simulink library "relay_ANSI_functions_lib"  (Simulink 8.1)
settings: Solver=ode45  StartTime=0.0  StopTime=10.0  RelTol=1e-3
undefined symbols (not defined in the file or in its folder): DiscIntNeverNeededParam, IOC, TOC, Ts, VRMSLL
libraries: simulink x8
settings Model: Creator=RE25624  LastModifiedBy=hptb1

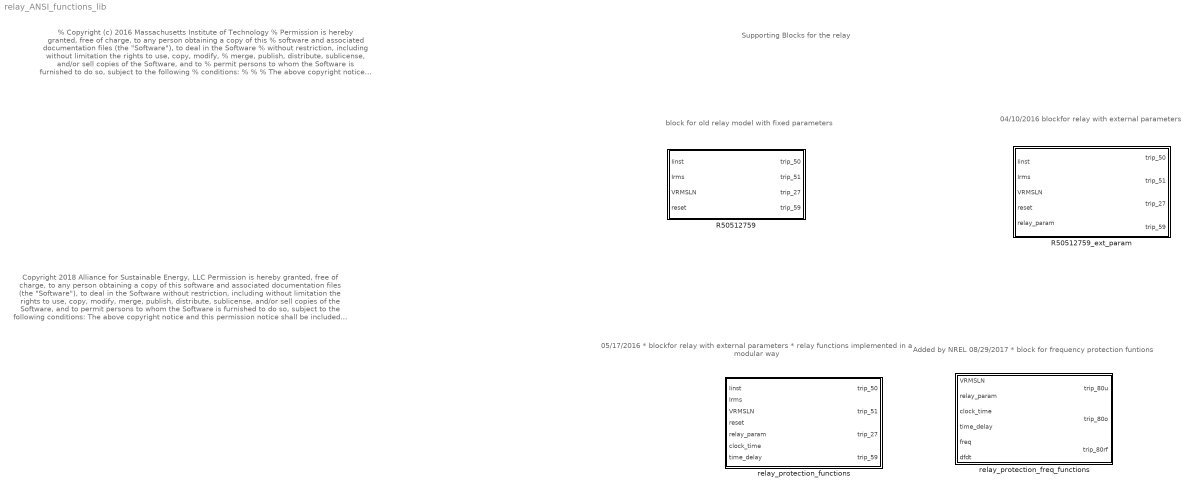
== system relay_ANSI_functions_lib ==
  note: 04/10/2016
      | blockfor relay with external parameters
  note: Supporting Blocks for the relay
  note: block for old relay model with fixed parameters
  note: 05/17/2016
      | * blockfor relay with external parameters
      | * relay functions implemented in a modular way
  note: % Copyright (c) 2016 Massachusetts Institute of Technology
      | % Permission is hereby granted, free of charge, to any person obtaining a copy of this
      | % software and associated documentation files (the "Software"), to deal in the Software
      | % without restriction, including without limitation the rights to use, copy, modify,
      | % merge, publish, distribute, sublicense, and/or sell copies of the Software, and to
      | % permit persons to whom the Software is furnished to do so, subject to the following
      | % conditions:
      | %
      | %
      | % The above copyright notice and this permission notice shall be included in
      | % all copies or substantial portions of the Software.
      | %
      | % THE SOFTWARE IS PROVIDED "AS IS", WITHOUT WARRANTY OF ANY KIND, EXPRESS OR IMPLIED,
      | % INCLUDING BUT NOT LIMITED TO THE WARRANTIES OF MERCHANTABILITY, FITNESS FOR A
      | % PARTICULAR PURPOSE AND NONINFRINGEMENT. IN NO EVENT SHALL THE AUTHORS OR COPYRIGHT
      | % HOLDERS BE LIABLE FOR ANY CLAIM, DAMAGES OR OTHER LIABILITY, WHETHER IN AN ACTION
      | % OF CONTRACT, TORT OR OTHERWISE, ARISING FROM, OUT OF OR IN CONNECTION WITH THE
      | % SOFTWARE OR THE USE OR OTHER DEALINGS IN THE SOFTWARE.
      | %
      | %
      | %%
  note: Added by NREL 08/29/2017
      | * block for frequency protection funtions
  note: Copyright 2018 Alliance for Sustainable Energy, LLC
      |
      | Permission is hereby granted, free of charge, to any person obtaining a copy of this software
      | and associated documentation files (the "Software"), to deal in the Software without restriction,
      | including without limitation the rights to use, copy, modify, merge, publish, distribute, sublicense,
      | and/or sell copies of the Software, and to permit persons to whom the Software is furnished to do so,
      | subject to the following conditions:
      |
      | The above copyright notice and this permission notice shall be included in all copies or substantial portions of the Software.
      |
      | THE SOFTWARE IS PROVIDED "AS IS", WITHOUT WARRANTY OF ANY KIND, EXPRESS OR IMPLIED, INCLUDING
      | BUT NOT LIMITED TO THE WARRANTIES OF MERCHANTABILITY, FITNESS FOR A PARTICULAR PURPOSE AND
      | NONINFRINGEMENT. IN NO EVENT SHALL THE AUTHORS, THE COPYRIGHT HOLDERS, THE UNITED STATES,
      | THE UNITED STATES DEPARTMENT OF ENERGY, OR ANY OF THEIR EMPLOYEES BE LIABLE FOR ANY CLAIM,
      | DAMAGES OR OTHER LIABILITY, WHETHER IN AN ACTION OF CONTRACT, TORT OR OTHERWISE, ARISING FROM,
      | OUT OF OR IN CONNECTION WITH THE SOFTWARE OR THE USE OR OTHER DEALINGS IN THE SOFTWARE.
  R50512759 : Subsystem  mask(Relays 50-51-27-59){VRMSLL=VRMSLL, IOC=IOC, TOC=TOC, Ts=Ts}
      mask prompts: VRMSLL "Nominal Voltage [VRMSLL]"; IOC "IOC Setting [A]"; TOC "TOC Setting [A]"; Ts "Sampling Time [Sec]"
      mask help:
      | This block simulates the behavior of the following relay functions:
      | 1) Instantaneous overcurrent (50)
      | 2) AC inverse time overcurrent (51)
      | 3) Undervoltage (27)
      | 4) Overvoltage (59)
      | It is not suitable for instantaneous earth current relaying.
      | The model neglects the influence CTs since only the logics of the relay are required or the current effort.
  R50512759_ext_param : Subsystem  mask(Relays 50-51-27-59){Ts=Ts}
      mask prompts: Ts "Sampling Time [Sec]"
      mask help:
      | This block simulates the behavior of the following relay functions:
      | 1) Instantaneous overcurrent (50)
      | 2) AC inverse time overcurrent (51)
      | 3) Undervoltage (27)
      | 4) Overvoltage (59)
      | It is not suitable for instantaneous earth current relaying.
      | The model neglects the influence CTs since only the logics of the relay are required or the current effort.
      |
      | The input bus with the relay parameters should be ordered as follows:
      | 1) VRMSLL
      | 2) IOC
      | 3) TOC
      | 4) dV_threshold
      | 5) angle_threshold
      | 6) dF_threshold
  relay_protection_freq_functions : Subsystem  mask(Relays 50-51-27-59){Ts=Ts}
      mask prompts: Ts "Sampling Time [Sec]"
      mask help:
      | This block simulates the behavior of the following relay functions:
      | 1)	Overfrequency (ANSI 81O)
      | 2)	Underfrequency (ANSI 81U)
      | 3)	Fast rate of change of frequency (ANSI 81R)
  relay_protection_functions : Subsystem  mask(Relays 50-51-27-59){Ts=Ts}
      mask prompts: Ts "Sampling Time [Sec]"
      mask help:
      | This block simulates the behavior of the following relay functions:
      | 1) Instantaneous overcurrent (50)
      | 2) AC inverse time overcurrent (51)
      | 3) Undervoltage (27)
      | 4) Overvoltage (59)
      | It is not suitable for instantaneous earth current relaying.
      | The model neglects the influence CTs since only the logics of the relay are required or the current effort.
      |
      | The input bus with the relay parameters should be ordered as follows:
      | 1) VRMSLL
      | 2) IOC
      | 3) TOC
      | 4) dV_threshold
      | 5) angle_threshold
      | 6) dF_threshold

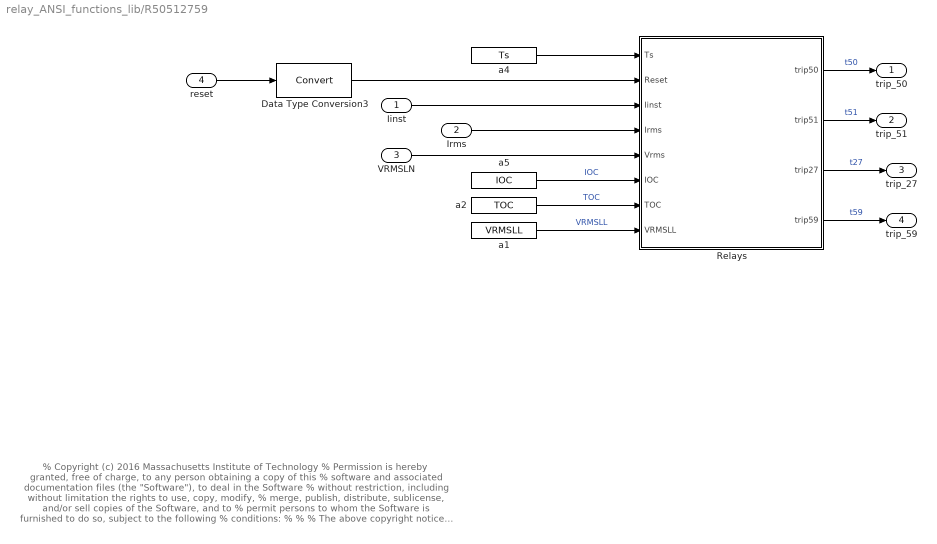
== system relay_ANSI_functions_lib/R50512759 ==
  note: % Copyright (c) 2016 Massachusetts Institute of Technology
      | % Permission is hereby granted, free of charge, to any person obtaining a copy of this
      | % software and associated documentation files (the "Software"), to deal in the Software
      | % without restriction, including without limitation the rights to use, copy, modify,
      | % merge, publish, distribute, sublicense, and/or sell copies of the Software, and to
      | % permit persons to whom the Software is furnished to do so, subject to the following
      | % conditions:
      | %
      | %
      | % The above copyright notice and this permission notice shall be included in
      | % all copies or substantial portions of the Software.
      | %
      | % THE SOFTWARE IS PROVIDED "AS IS", WITHOUT WARRANTY OF ANY KIND, EXPRESS OR IMPLIED,
      | % INCLUDING BUT NOT LIMITED TO THE WARRANTIES OF MERCHANTABILITY, FITNESS FOR A
      | % PARTICULAR PURPOSE AND NONINFRINGEMENT. IN NO EVENT SHALL THE AUTHORS OR COPYRIGHT
      | % HOLDERS BE LIABLE FOR ANY CLAIM, DAMAGES OR OTHER LIABILITY, WHETHER IN AN ACTION
      | % OF CONTRACT, TORT OR OTHERWISE, ARISING FROM, OUT OF OR IN CONNECTION WITH THE
      | % SOFTWARE OR THE USE OR OTHER DEALINGS IN THE SOFTWARE.
      | %
      | %
      | %%
  Iinst : Inport
  Irms : Inport  Port=2
  VRMSLN : Inport  Port=3
  reset : Inport  Port=4
  Data Type Conversion3 : DataTypeConversion
  Relays : MATLAB Function  TreatAsAtomicUnit=on
  a1 : Constant  Value=VRMSLL
  a2 : Constant  Value=TOC
  a4 : Constant  Value=Ts
  a5 : Constant  Value=IOC
  trip_50 : Outport
  trip_51 : Outport  Port=2
  trip_27 : Outport  Port=3
  trip_59 : Outport  Port=4
  wires:
  Data Type Conversion3/1 -> Relays/2(Reset)
  Relays/2(trip51) -> trip_51/1  "t51"
  Relays/1(trip50) -> trip_50/1  "t50"
  Relays/4(trip59) -> trip_59/1  "t59"
  Relays/3(trip27) -> trip_27/1  "t27"
  a4/1 -> Relays/1(Ts)
  a1/1 -> Relays/8(VRMSLL)  "VRMSLL"
  VRMSLN/1 -> Relays/5(Vrms)
  Irms/1 -> Relays/4(Irms)
  a2/1 -> Relays/7(TOC)  "TOC"
  Iinst/1 -> Relays/3(Iinst)
  a5/1 -> Relays/6(IOC)  "IOC"
  reset/1 -> Data Type Conversion3/1

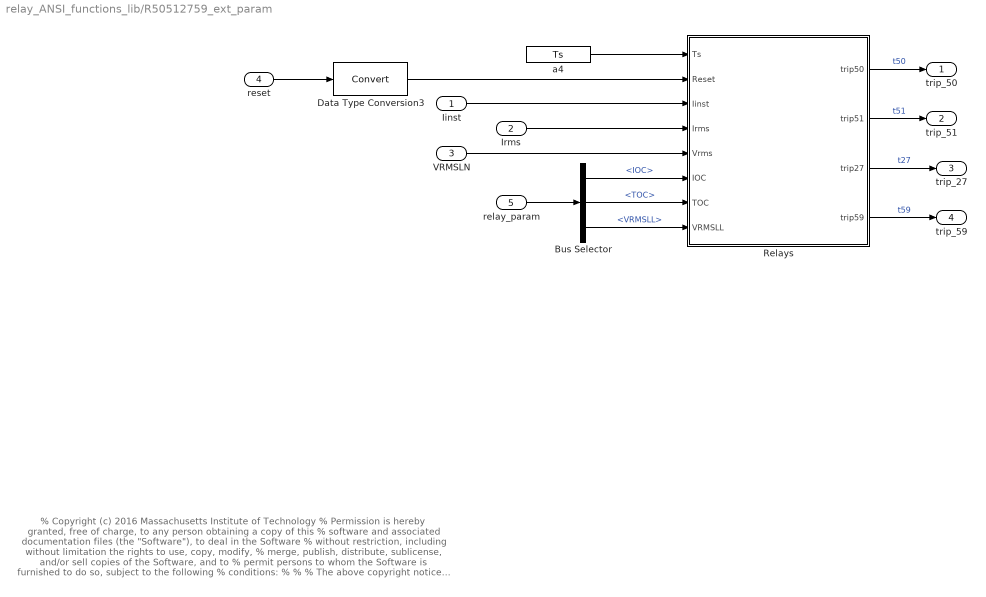
== system relay_ANSI_functions_lib/R50512759_ext_param ==
  note: % Copyright (c) 2016 Massachusetts Institute of Technology
      | % Permission is hereby granted, free of charge, to any person obtaining a copy of this
      | % software and associated documentation files (the "Software"), to deal in the Software
      | % without restriction, including without limitation the rights to use, copy, modify,
      | % merge, publish, distribute, sublicense, and/or sell copies of the Software, and to
      | % permit persons to whom the Software is furnished to do so, subject to the following
      | % conditions:
      | %
      | %
      | % The above copyright notice and this permission notice shall be included in
      | % all copies or substantial portions of the Software.
      | %
      | % THE SOFTWARE IS PROVIDED "AS IS", WITHOUT WARRANTY OF ANY KIND, EXPRESS OR IMPLIED,
      | % INCLUDING BUT NOT LIMITED TO THE WARRANTIES OF MERCHANTABILITY, FITNESS FOR A
      | % PARTICULAR PURPOSE AND NONINFRINGEMENT. IN NO EVENT SHALL THE AUTHORS OR COPYRIGHT
      | % HOLDERS BE LIABLE FOR ANY CLAIM, DAMAGES OR OTHER LIABILITY, WHETHER IN AN ACTION
      | % OF CONTRACT, TORT OR OTHERWISE, ARISING FROM, OUT OF OR IN CONNECTION WITH THE
      | % SOFTWARE OR THE USE OR OTHER DEALINGS IN THE SOFTWARE.
      | %
      | %
      | %%
  Iinst : Inport
  Irms : Inport  Port=2
  VRMSLN : Inport  Port=3
  reset : Inport  Port=4
  relay_param : Inport  Port=5
  Bus Selector : BusSelector  OutputSignals=IOC,TOC,VRMSLL
  Data Type Conversion3 : DataTypeConversion
  Relays : MATLAB Function  TreatAsAtomicUnit=on
  a4 : Constant  Value=Ts
  trip_50 : Outport
  trip_51 : Outport  Port=2
  trip_27 : Outport  Port=3
  trip_59 : Outport  Port=4
  wires:
  relay_param/1 -> Bus Selector/1
  Data Type Conversion3/1 -> Relays/2(Reset)
  Relays/2(trip51) -> trip_51/1  "t51"
  Relays/1(trip50) -> trip_50/1  "t50"
  Relays/4(trip59) -> trip_59/1  "t59"
  Relays/3(trip27) -> trip_27/1  "t27"
  a4/1 -> Relays/1(Ts)
  Bus Selector/3 -> Relays/8(VRMSLL)  "<VRMSLL>"
  VRMSLN/1 -> Relays/5(Vrms)
  Irms/1 -> Relays/4(Irms)
  Bus Selector/2 -> Relays/7(TOC)  "<TOC>"
  Iinst/1 -> Relays/3(Iinst)
  Bus Selector/1 -> Relays/6(IOC)  "<IOC>"
  reset/1 -> Data Type Conversion3/1

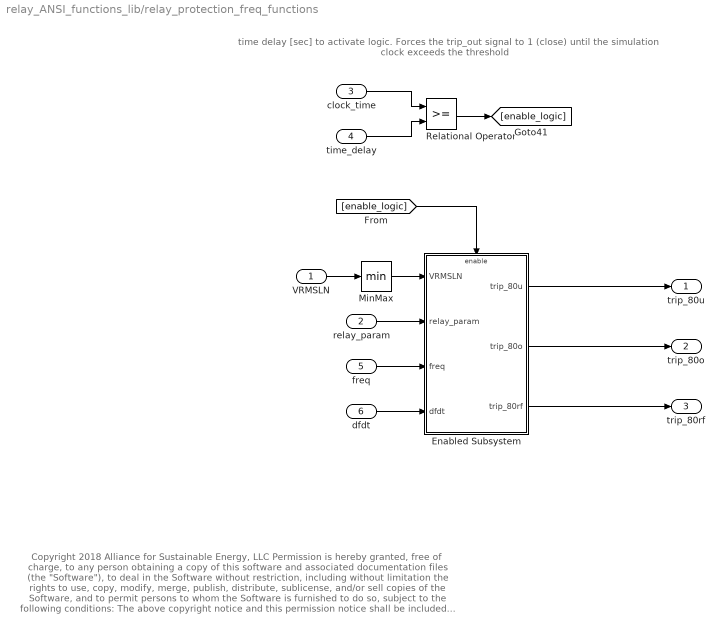
== system relay_ANSI_functions_lib/relay_protection_freq_functions ==
  note: Copyright 2018 Alliance for Sustainable Energy, LLC
      |
      | Permission is hereby granted, free of charge, to any person obtaining a copy of this software
      | and associated documentation files (the "Software"), to deal in the Software without restriction,
      | including without limitation the rights to use, copy, modify, merge, publish, distribute, sublicense,
      | and/or sell copies of the Software, and to permit persons to whom the Software is furnished to do so,
      | subject to the following conditions:
      |
      | The above copyright notice and this permission notice shall be included in all copies or substantial portions of the Software.
      |
      | THE SOFTWARE IS PROVIDED "AS IS", WITHOUT WARRANTY OF ANY KIND, EXPRESS OR IMPLIED, INCLUDING
      | BUT NOT LIMITED TO THE WARRANTIES OF MERCHANTABILITY, FITNESS FOR A PARTICULAR PURPOSE AND
      | NONINFRINGEMENT. IN NO EVENT SHALL THE AUTHORS, THE COPYRIGHT HOLDERS, THE UNITED STATES,
      | THE UNITED STATES DEPARTMENT OF ENERGY, OR ANY OF THEIR EMPLOYEES BE LIABLE FOR ANY CLAIM,
      | DAMAGES OR OTHER LIABILITY, WHETHER IN AN ACTION OF CONTRACT, TORT OR OTHERWISE, ARISING FROM,
      | OUT OF OR IN CONNECTION WITH THE SOFTWARE OR THE USE OR OTHER DEALINGS IN THE SOFTWARE.
  note: time delay [sec] to activate logic. Forces the trip_out signal
      | to 1 (close) until the simulation clock exceeds the threshold
  VRMSLN : Inport
  relay_param : Inport  Port=2
  clock_time : Inport  Port=3
  time_delay : Inport  Port=4
  freq : Inport  Port=5
  dfdt : Inport  Port=6
  Enabled Subsystem : Subsystem  TreatAsAtomicUnit=on
  MinMax : MinMax
  Relational Operator : RelationalOperator  OutDataTypeStr=boolean
  trip_80u : Outport
  trip_80o : Outport  Port=2
  trip_80rf : Outport  Port=3
  wires:
  [enable_logic] -> Enabled Subsystem/Enable
  Relational Operator/1 -> [enable_logic]
  time_delay/1 -> Relational Operator/2
  clock_time/1 -> Relational Operator/1
  VRMSLN/1 -> MinMax/1
  Enabled Subsystem/1(trip_80u) -> trip_80u/1
  Enabled Subsystem/2(trip_80o) -> trip_80o/1
  Enabled Subsystem/3(trip_80rf) -> trip_80rf/1
  relay_param/1 -> Enabled Subsystem/2(relay_param)
  freq/1 -> Enabled Subsystem/3(freq)
  dfdt/1 -> Enabled Subsystem/4(dfdt)
  MinMax/1 -> Enabled Subsystem/1(VRMSLN)

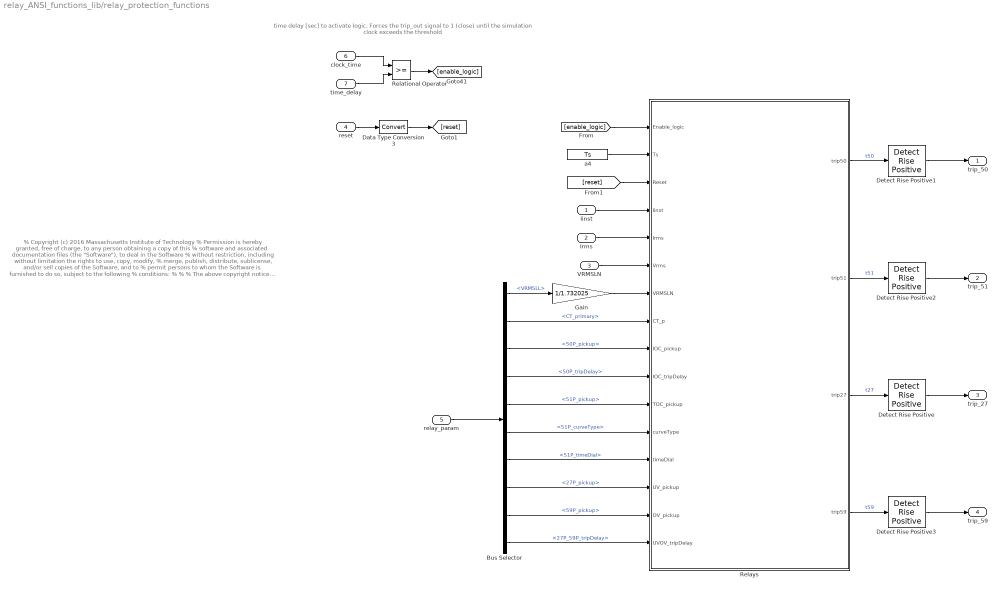
== system relay_ANSI_functions_lib/relay_protection_functions ==
  note: % Copyright (c) 2016 Massachusetts Institute of Technology
      | % Permission is hereby granted, free of charge, to any person obtaining a copy of this
      | % software and associated documentation files (the "Software"), to deal in the Software
      | % without restriction, including without limitation the rights to use, copy, modify,
      | % merge, publish, distribute, sublicense, and/or sell copies of the Software, and to
      | % permit persons to whom the Software is furnished to do so, subject to the following
      | % conditions:
      | %
      | %
      | % The above copyright notice and this permission notice shall be included in
      | % all copies or substantial portions of the Software.
      | %
      | % THE SOFTWARE IS PROVIDED "AS IS", WITHOUT WARRANTY OF ANY KIND, EXPRESS OR IMPLIED,
      | % INCLUDING BUT NOT LIMITED TO THE WARRANTIES OF MERCHANTABILITY, FITNESS FOR A
      | % PARTICULAR PURPOSE AND NONINFRINGEMENT. IN NO EVENT SHALL THE AUTHORS OR COPYRIGHT
      | % HOLDERS BE LIABLE FOR ANY CLAIM, DAMAGES OR OTHER LIABILITY, WHETHER IN AN ACTION
      | % OF CONTRACT, TORT OR OTHERWISE, ARISING FROM, OUT OF OR IN CONNECTION WITH THE
      | % SOFTWARE OR THE USE OR OTHER DEALINGS IN THE SOFTWARE.
      | %
      | %
      | %%
  note: time delay [sec] to activate logic. Forces the trip_out signal
      | to 1 (close) until the simulation clock exceeds the threshold
  Iinst : Inport
  Irms : Inport  Port=2
  VRMSLN : Inport  Port=3
  reset : Inport  Port=4
  relay_param : Inport  Port=5
  clock_time : Inport  Port=6
  time_delay : Inport  Port=7
  Bus Selector : BusSelector  OutputSignals=VRMSLL,CT_primary,50P_pickup,50P_tripDelay,51P_pickup,51P_curveType,51P_timeDial,27P_pickup,59P_pickup,27P_59P_tripDelay
  Data Type Conversion3 : DataTypeConversion
  Detect Rise Positive{,1..3} (4 alike) : simulink/Logic and Bit Operations/Detect Rise Positive  vinit=0  InputProcessing=Inherited  OutDataTypeStr=boolean
  Gain : Gain  Gain=1/1.732025
  Relational Operator : RelationalOperator  OutDataTypeStr=boolean
  Relays : MATLAB Function  TreatAsAtomicUnit=on
  a4 : Constant  Value=Ts
  trip_50 : Outport
  trip_51 : Outport  Port=2
  trip_27 : Outport  Port=3
  trip_59 : Outport  Port=4
  wires:
  [enable_logic] -> Relays/1(Enable_logic)
  Relational Operator/1 -> [enable_logic]
  time_delay/1 -> Relational Operator/2
  clock_time/1 -> Relational Operator/1
  relay_param/1 -> Bus Selector/1
  a4/1 -> Relays/2(Ts)
  VRMSLN/1 -> Relays/6(Vrms)
  reset/1 -> Data Type Conversion3/1
  Bus Selector/1 -> Gain/1  "<VRMSLL>"
  Bus Selector/2 -> Relays/8(CT_p)  "<CT_primary>"
  Bus Selector/3 -> Relays/9(IOC_pickup)  "<50P_pickup>"
  Bus Selector/4 -> Relays/10(IOC_tripDelay)  "<50P_tripDelay>"
  Bus Selector/5 -> Relays/11(TOC_pickup)  "<51P_pickup>"
  Bus Selector/6 -> Relays/12(curveType)  "<51P_curveType>"
  Bus Selector/7 -> Relays/13(timeDial)  "<51P_timeDial>"
  Irms/1 -> Relays/5(Irms)
  Iinst/1 -> Relays/4(Iinst)
  Bus Selector/10 -> Relays/16(UVOV_tripDelay)  "<27P_59P_tripDelay>"
  Bus Selector/9 -> Relays/15(OV_pickup)  "<59P_pickup>"
  Bus Selector/8 -> Relays/14(UV_pickup)  "<27P_pickup>"
  Gain/1 -> Relays/7(VRMSLN)
  Data Type Conversion3/1 -> [reset]
  [reset] -> Relays/3(Reset)
  Relays/3(trip27) -> Detect Rise Positive/1  "t27"
  Relays/1(trip50) -> Detect Rise Positive1/1  "t50"
  Relays/2(trip51) -> Detect Rise Positive2/1  "t51"
  Relays/4(trip59) -> Detect Rise Positive3/1  "t59"
  Detect Rise Positive1/1 -> trip_50/1
  Detect Rise Positive2/1 -> trip_51/1
  Detect Rise Positive/1 -> trip_27/1
  Detect Rise Positive3/1 -> trip_59/1

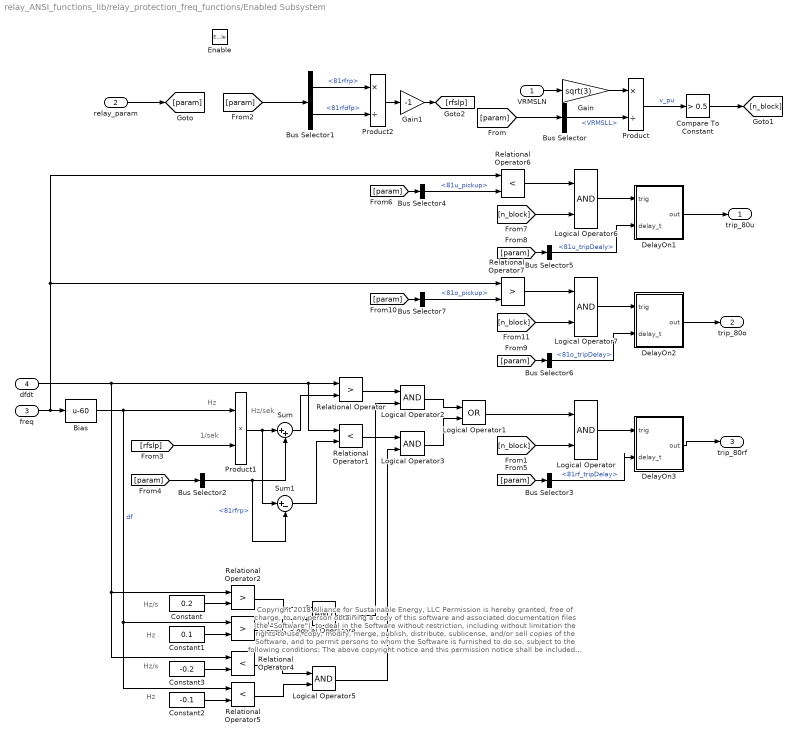
== system relay_ANSI_functions_lib/relay_protection_freq_functions/Enabled Subsystem ==
  note: Copyright 2018 Alliance for Sustainable Energy, LLC
      |
      | Permission is hereby granted, free of charge, to any person obtaining a copy of this software
      | and associated documentation files (the "Software"), to deal in the Software without restriction,
      | including without limitation the rights to use, copy, modify, merge, publish, distribute, sublicense,
      | and/or sell copies of the Software, and to permit persons to whom the Software is furnished to do so,
      | subject to the following conditions:
      |
      | The above copyright notice and this permission notice shall be included in all copies or substantial portions of the Software.
      |
      | THE SOFTWARE IS PROVIDED "AS IS", WITHOUT WARRANTY OF ANY KIND, EXPRESS OR IMPLIED, INCLUDING
      | BUT NOT LIMITED TO THE WARRANTIES OF MERCHANTABILITY, FITNESS FOR A PARTICULAR PURPOSE AND
      | NONINFRINGEMENT. IN NO EVENT SHALL THE AUTHORS, THE COPYRIGHT HOLDERS, THE UNITED STATES,
      | THE UNITED STATES DEPARTMENT OF ENERGY, OR ANY OF THEIR EMPLOYEES BE LIABLE FOR ANY CLAIM,
      | DAMAGES OR OTHER LIABILITY, WHETHER IN AN ACTION OF CONTRACT, TORT OR OTHERWISE, ARISING FROM,
      | OUT OF OR IN CONNECTION WITH THE SOFTWARE OR THE USE OR OTHER DEALINGS IN THE SOFTWARE.
  note: Hz
  note: Hz/sek
  note: 1/sek
  note: Hz
  note: Hz
  note: Hz/s
  note: Hz/s
  VRMSLN : Inport
  relay_param : Inport  Port=2
  freq : Inport  Port=3
  dfdt : Inport  Port=4
  Enable : EnablePort
  Bias : Bias  Bias=-60
  Bus Selector : BusSelector  OutputSignals=VRMSLL
  Bus Selector1 : BusSelector  OutputSignals=81rfrp,81rfdfp
  Bus Selector2 : BusSelector  OutputSignals=81rfrp
  Bus Selector3 : BusSelector  OutputSignals=81rf_tripDelay
  Bus Selector4 : BusSelector  OutputSignals=81u_pickup
  Bus Selector5 : BusSelector  OutputSignals=81u_tripDealy
  Bus Selector6 : BusSelector  OutputSignals=81o_tripDelay
  Bus Selector7 : BusSelector  OutputSignals=81o_pickup
  Compare To Constant : simulink/Logic and Bit Operations/Compare To Constant  relop=>  const=0.5  OutDataTypeStr=boolean
  Constant : Constant  Value=0.2
  Constant1 : Constant  Value=0.1
  Constant2 : Constant  Value=-0.1
  Constant3 : Constant  Value=-0.2
  DelayOn1 : Subsystem
  DelayOn2 : Subsystem
  DelayOn3 : Subsystem
  Gain : Gain  Gain=sqrt(3)
  Gain1 : Gain  Gain=-1
  Logical Operator{,2..7} (7 alike) : Logic  AllPortsSameDT=off  OutDataTypeStr=boolean
  Logical Operator1 : Logic  Operator=OR  AllPortsSameDT=off  OutDataTypeStr=boolean
  Product : Product  Inputs=*/
  Product1 : Product
  Product2 : Product  Inputs=*/
  Relational Operator{,2..3,7} (4 alike) : RelationalOperator  Operator=>  OutDataTypeStr=boolean
  Relational Operator{1,4..6} (4 alike) : RelationalOperator  Operator=<  OutDataTypeStr=boolean
  Sum : Sum  Inputs=|++
  Sum1 : Sum  Inputs=|+-
  trip_80u : Outport
  trip_80o : Outport  Port=2
  trip_80rf : Outport  Port=3
  wires:
  relay_param/1 -> [param]
  [param] -> Bus Selector/1
  VRMSLN/1 -> Gain/1
  Bus Selector/1 -> Product/2  "<VRMSLL>"
  Product/1 -> Compare To Constant/1  "v_pu"
  Gain/1 -> Product/1
  Compare To Constant/1 -> [n_block]
  [n_block] -> Logical Operator/2
  Logical Operator1/1 -> Logical Operator/1
  dfdt/1 -> Relational Operator4/1, Relational Operator2/1, Relational Operator/1, Relational Operator1/1
  [param] -> Bus Selector1/1
  Bus Selector1/1 -> Product2/1  "<81rfrp>"
  freq/1 -> Relational Operator7/1, Relational Operator6/1, Bias/1
  Sum1/1 -> Relational Operator1/2
  Bias/1 -> Relational Operator5/1, Relational Operator3/1, Product1/1  "df"
  [rfslp] -> Product1/2
  Bus Selector1/2 -> Product2/2  "<81rfdfp>"
  Product2/1 -> Gain1/1
  Product1/1 -> Sum1/1, Sum/1
  [param] -> Bus Selector2/1
  Bus Selector2/1 -> Sum/2, Sum1/2  "<81rfrp>"
  Sum/1 -> Relational Operator/2
  Relational Operator/1 -> Logical Operator2/1
  Relational Operator1/1 -> Logical Operator3/1
  Logical Operator2/1 -> Logical Operator1/1
  Logical Operator3/1 -> Logical Operator1/2
  Logical Operator4/1 -> Logical Operator2/2
  Logical Operator5/1 -> Logical Operator3/2
  Relational Operator2/1 -> Logical Operator4/1
  Relational Operator3/1 -> Logical Operator4/2
  Relational Operator4/1 -> Logical Operator5/1
  Relational Operator5/1 -> Logical Operator5/2
  Constant/1 -> Relational Operator2/2
  Constant1/1 -> Relational Operator3/2
  Constant3/1 -> Relational Operator4/2
  Constant2/1 -> Relational Operator5/2
  [param] -> Bus Selector3/1
  Logical Operator/1 -> DelayOn3/1(trig)
  Bus Selector3/1 -> DelayOn3/2(delay_t)  "<81rf_tripDelay>"
  DelayOn3/1(out) -> trip_80rf/1
  DelayOn2/1(out) -> trip_80o/1
  DelayOn1/1(out) -> trip_80u/1
  [param] -> Bus Selector4/1
  Bus Selector4/1 -> Relational Operator6/2  "<81u_pickup>"
  [n_block] -> Logical Operator6/2
  Logical Operator6/1 -> DelayOn1/1(trig)
  Relational Operator6/1 -> Logical Operator6/1
  [param] -> Bus Selector5/1
  Bus Selector5/1 -> DelayOn1/2(delay_t)  "<81u_tripDealy>"
  [param] -> Bus Selector6/1
  Bus Selector6/1 -> DelayOn2/2(delay_t)  "<81o_tripDelay>"
  [param] -> Bus Selector7/1
  Bus Selector7/1 -> Relational Operator7/2  "<81o_pickup>"
  [n_block] -> Logical Operator7/2
  Relational Operator7/1 -> Logical Operator7/1
  Logical Operator7/1 -> DelayOn2/1(trig)
  Gain1/1 -> [rfslp]

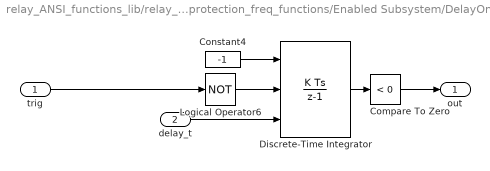
== system relay_ANSI_functions_lib/relay_protection_freq_functions/Enabled Subsystem/DelayOn1 ==
  trig : Inport
  delay_t : Inport  Port=2
  Compare To Zero : simulink/Logic and Bit Operations/Compare To Zero  relop=<  OutDataTypeStr=boolean
  Constant4 : Constant  Value=-1
  Discrete-Time Integrator : DiscreteIntegrator  ExternalReset=level  InitialConditionSource=external  SampleTime=Ts  LimitOutput=on  LowerSaturationLimit=-1  ICPrevOutput=DiscIntNeverNeededParam  ICPrevScaledInput=DiscIntNeverNeededParam
  Logical Operator6 : Logic  Operator=NOT  AllPortsSameDT=off  OutDataTypeStr=boolean
  out : Outport
  wires:
  Logical Operator6/1 -> Discrete-Time Integrator/2
  delay_t/1 -> Discrete-Time Integrator/3
  Discrete-Time Integrator/1 -> Compare To Zero/1
  Constant4/1 -> Discrete-Time Integrator/1
  Compare To Zero/1 -> out/1
  trig/1 -> Logical Operator6/1

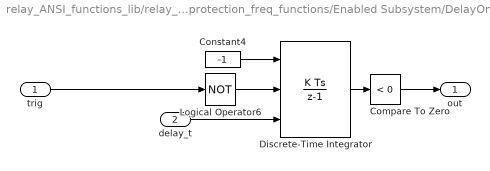
== system relay_ANSI_functions_lib/relay_protection_freq_functions/Enabled Subsystem/DelayOn2 ==
  trig : Inport
  delay_t : Inport  Port=2
  Compare To Zero : simulink/Logic and Bit Operations/Compare To Zero  relop=<  OutDataTypeStr=boolean
  Constant4 : Constant  Value=-1
  Discrete-Time Integrator : DiscreteIntegrator  ExternalReset=level  InitialConditionSource=external  SampleTime=Ts  LimitOutput=on  LowerSaturationLimit=-1  ICPrevOutput=DiscIntNeverNeededParam  ICPrevScaledInput=DiscIntNeverNeededParam
  Logical Operator6 : Logic  Operator=NOT  AllPortsSameDT=off  OutDataTypeStr=boolean
  out : Outport
  wires:
  trig/1 -> Logical Operator6/1
  Compare To Zero/1 -> out/1
  Constant4/1 -> Discrete-Time Integrator/1
  Discrete-Time Integrator/1 -> Compare To Zero/1
  delay_t/1 -> Discrete-Time Integrator/3
  Logical Operator6/1 -> Discrete-Time Integrator/2

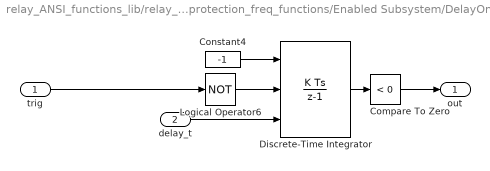
== system relay_ANSI_functions_lib/relay_protection_freq_functions/Enabled Subsystem/DelayOn3 ==
  trig : Inport
  delay_t : Inport  Port=2
  Compare To Zero : simulink/Logic and Bit Operations/Compare To Zero  relop=<  OutDataTypeStr=boolean
  Constant4 : Constant  Value=-1
  Discrete-Time Integrator : DiscreteIntegrator  ExternalReset=level  InitialConditionSource=external  SampleTime=Ts  LimitOutput=on  LowerSaturationLimit=-1  ICPrevOutput=DiscIntNeverNeededParam  ICPrevScaledInput=DiscIntNeverNeededParam
  Logical Operator6 : Logic  Operator=NOT  AllPortsSameDT=off  OutDataTypeStr=boolean
  out : Outport
  wires:
  trig/1 -> Logical Operator6/1
  Compare To Zero/1 -> out/1
  Constant4/1 -> Discrete-Time Integrator/1
  Discrete-Time Integrator/1 -> Compare To Zero/1
  delay_t/1 -> Discrete-Time Integrator/3
  Logical Operator6/1 -> Discrete-Time Integrator/2

== matlab function relay_protection_functions/Relays ==
  data: Enable_logic input double; Ts input double; Reset input double; Iinst input double; Irms input double; Vrms input double; VRMSLN input double; CT_p input double; IOC_pickup input double; IOC_tripDelay input double; TOC_pickup input double; curveType input double; timeDial input double; UV_pickup input double; OV_pickup input double; UVOV_tripDelay input double; trip50 output double; trip51 output double; trip27 output double; trip59 output double
% Copyright (c) 2016 Massachusetts Institute of Technology
% Permission is hereby granted, free of charge, to any person obtaining a copy of this
% software and associated documentation files (the "Software"), to deal in the Software
% without restriction, including without limitation the rights to use, copy, modify,
% merge, publish, distribute, sublicense, and/or sell copies of the Software, and to
% permit persons to whom the Software is furnished to do so, subject to the following
% conditions:
%
%
% The above copyright notice and this permission notice shall be included in
% all copies or substantial portions of the Software.
%
% THE SOFTWARE IS PROVIDED "AS IS", WITHOUT WARRANTY OF ANY KIND, EXPRESS OR IMPLIED,
% INCLUDING BUT NOT LIMITED TO THE WARRANTIES OF MERCHANTABILITY, FITNESS FOR A
% PARTICULAR PURPOSE AND NONINFRINGEMENT. IN NO EVENT SHALL THE AUTHORS OR COPYRIGHT
% HOLDERS BE LIABLE FOR ANY CLAIM, DAMAGES OR OTHER LIABILITY, WHETHER IN AN ACTION
% OF CONTRACT, TORT OR OTHERWISE, ARISING FROM, OUT OF OR IN CONNECTION WITH THE
% SOFTWARE OR THE USE OR OTHER DEALINGS IN THE SOFTWARE.
%
%
%%

function [trip50, trip51, trip27, trip59] = relay_elements(Enable_logic, Ts, Reset, Iinst, Irms, Vrms, VRMSLN,...
    CT_p, IOC_pickup, IOC_tripDelay, TOC_pickup, curveType, timeDial, UV_pickup, OV_pickup, UVOV_tripDelay)
%#codegen

% initialize or reset the trip signals
persistent R50 R51 R27 R59
if isempty(R51) || Reset
    R50=false;
    R51=false;
    R59=false;
    R27=false;
end

% applying turns CT ratio - assuming protection type CT
Iinst = Iinst * (5/CT_p);
Irms = Irms * (5/CT_p);

% old- latch for true signals
% old- if ~(R50==true || R51==true) && Enable_logic==1
if Enable_logic==1
    % calling external function expressing relay protection elements
    T50 = relay_ANSI_50P_script(Ts, Iinst , IOC_pickup, IOC_tripDelay);
    T51 = relay_ANSI_51P_script(Ts, Irms, TOC_pickup, curveType, timeDial);
    T27 = relay_ANSI_27P_script(Ts, Vrms, VRMSLN, UV_pickup, UVOV_tripDelay);
    T59 = relay_ANSI_59P_script(Ts, Vrms, VRMSLN, OV_pickup, UVOV_tripDelay);
    
    R50 = T50;
    R51 = T51;
    R27 = T27;
    R59 = T59;
end

% external latch
trip50 = R50; % old- latched
trip51 = R51; % old- latched
trip27 = R27; % old- not latched
trip59 = R59; % old- not latched

== matlab function R50512759/Relays ==
  data: Ts input double; trip50 output double; Reset input double; Iinst input double; Irms input double; Vrms input double; IOC input double; trip51 output double; trip27 output double; TOC input double; VRMSLL input double; trip59 output double
% Copyright (c) 2016 Massachusetts Institute of Technology
% Permission is hereby granted, free of charge, to any person obtaining a copy of this 
% software and associated documentation files (the "Software"), to deal in the Software
% without restriction, including without limitation the rights to use, copy, modify, 
% merge, publish, distribute, sublicense, and/or sell copies of the Software, and to 
% permit persons to whom the Software is furnished to do so, subject to the following 
% conditions:
% 
% 
% The above copyright notice and this permission notice shall be included in 
% all copies or substantial portions of the Software.
% 
% THE SOFTWARE IS PROVIDED "AS IS", WITHOUT WARRANTY OF ANY KIND, EXPRESS OR IMPLIED, 
% INCLUDING BUT NOT LIMITED TO THE WARRANTIES OF MERCHANTABILITY, FITNESS FOR A 
% PARTICULAR PURPOSE AND NONINFRINGEMENT. IN NO EVENT SHALL THE AUTHORS OR COPYRIGHT 
% HOLDERS BE LIABLE FOR ANY CLAIM, DAMAGES OR OTHER LIABILITY, WHETHER IN AN ACTION 
% OF CONTRACT, TORT OR OTHERWISE, ARISING FROM, OUT OF OR IN CONNECTION WITH THE 
% SOFTWARE OR THE USE OR OTHER DEALINGS IN THE SOFTWARE.
%
%
%%


function [trip50, trip51, trip27, trip59] = relays_50512759(Ts, Reset, Iinst, Irms, Vrms, IOC, TOC, VRMSLL)
%#codegen

% initialize or reset the trip signals
persistent R50 R51 R27 R59
if isempty(R51) || Reset
    R50=false;
    R51=false;
    R59=false;
    R27=false;
end

% latch for true signals
if ~(R50==true || R51==true)
    % calling external function
    r = relay_ANSI_50512759_script(Ts, Iinst, Irms, Vrms, IOC, TOC, VRMSLL);
    R50 = r.trip50;
    R51 = r.trip51;
    R27 = r.trip27;
    R59 = r.trip59;
end

trip50 = R50; % latched
trip51 = R51; % latched
trip27 = R27; % not latched
trip59 = R59; % not latched

== matlab function R50512759_ext_param/Relays ==
  data: Ts input double; trip50 output double; Reset input double; Iinst input double; Irms input double; Vrms input double; IOC input double; trip51 output double; trip27 output double; TOC input double; VRMSLL input double; trip59 output double
% Copyright (c) 2016 Massachusetts Institute of Technology
% Permission is hereby granted, free of charge, to any person obtaining a copy of this 
% software and associated documentation files (the "Software"), to deal in the Software
% without restriction, including without limitation the rights to use, copy, modify, 
% merge, publish, distribute, sublicense, and/or sell copies of the Software, and to 
% permit persons to whom the Software is furnished to do so, subject to the following 
% conditions:
% 
% 
% The above copyright notice and this permission notice shall be included in 
% all copies or substantial portions of the Software.
% 
% THE SOFTWARE IS PROVIDED "AS IS", WITHOUT WARRANTY OF ANY KIND, EXPRESS OR IMPLIED, 
% INCLUDING BUT NOT LIMITED TO THE WARRANTIES OF MERCHANTABILITY, FITNESS FOR A 
% PARTICULAR PURPOSE AND NONINFRINGEMENT. IN NO EVENT SHALL THE AUTHORS OR COPYRIGHT 
% HOLDERS BE LIABLE FOR ANY CLAIM, DAMAGES OR OTHER LIABILITY, WHETHER IN AN ACTION 
% OF CONTRACT, TORT OR OTHERWISE, ARISING FROM, OUT OF OR IN CONNECTION WITH THE 
% SOFTWARE OR THE USE OR OTHER DEALINGS IN THE SOFTWARE.
%
%
%%

function [trip50, trip51, trip27, trip59] = relays_50512759(Ts, Reset, Iinst, Irms, Vrms, IOC, TOC, VRMSLL)
%#codegen

% initialize or reset the trip signals
persistent R50 R51 R27 R59
if isempty(R51) || Reset
    R50=false;
    R51=false;
    R59=false;
    R27=false;
end

% latch for true signals
if ~(R50==true || R51==true)
    % calling external function
    r = relay_ANSI_50512759_script(Ts, Iinst, Irms, Vrms, IOC, TOC, VRMSLL);
    R50 = r.trip50;
    R51 = r.trip51;
    R27 = r.trip27;
    R59 = r.trip59;
end

trip50 = R50; % latched
trip51 = R51; % latched
trip27 = R27; % not latched
trip59 = R59; % not latched
